simulink model "SYT_A23_mod"  (Simulink 5.1)
settings: Solver=ode5  SolverMode=SingleTasking  StartTime=0.0  StopTime=20.0  FixedStep=0.1  RelTol=1e-3
settings Model: LastModifiedBy=Sommer  BooleanDataType=on  ProdHWDeviceType=Microprocessor

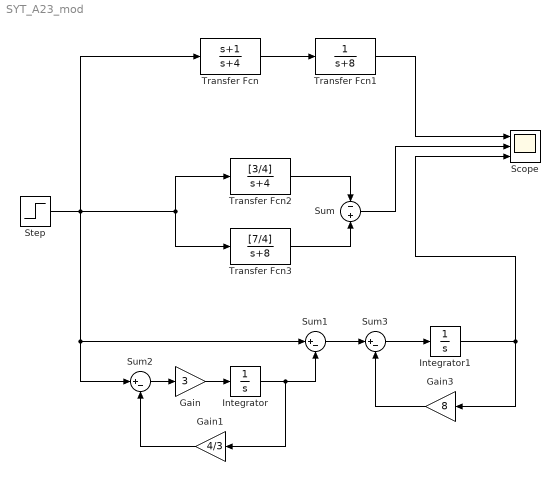
== system SYT_A23_mod ==
  Gain : Gain  Gain=3  SaturateOnIntegerOverflow=on
  Gain1 : Gain  Orientation=left  Gain=4/3  SaturateOnIntegerOverflow=on
  Gain3 : Gain  Orientation=left  Gain=8  SaturateOnIntegerOverflow=on
  Integrator : Integrator
  Integrator1 : Integrator
  Scope : Scope  NumInputPorts=3
      settings: YMin=-5~-5~-5  YMax=5~5~5
  Step : Step  SampleTime=0
  Sum : Sum  Inputs=-|+  SaturateOnIntegerOverflow=on  InputSameDT=on
  Sum1 : Sum  Inputs=|+-  SaturateOnIntegerOverflow=on  InputSameDT=on
  Sum2 : Sum  Inputs=|+-  SaturateOnIntegerOverflow=on  InputSameDT=on
  Sum3 : Sum  Inputs=|+-  SaturateOnIntegerOverflow=on  InputSameDT=on
  Transfer Fcn : TransferFcn  Numerator=[1 1]  Denominator=[1 4]
  Transfer Fcn1 : TransferFcn  Denominator=[1 8]
  Transfer Fcn2 : TransferFcn  Numerator=[3/4]  Denominator=[1 4]
  Transfer Fcn3 : TransferFcn  Numerator=[7/4]  Denominator=[1 8]
  wires:
  Transfer Fcn/1 -> Transfer Fcn1/1
  Step/1 -> Transfer Fcn/1, Transfer Fcn2/1, Transfer Fcn3/1, Sum2/1, Sum1/1
  Transfer Fcn1/1 -> Scope/1
  Transfer Fcn2/1 -> Sum/1
  Transfer Fcn3/1 -> Sum/2
  Sum/1 -> Scope/2
  Gain/1 -> Integrator/1
  Gain1/1 -> Sum2/2
  Sum2/1 -> Gain/1
  Integrator/1 -> Sum1/2, Gain1/1
  Sum3/1 -> Integrator1/1
  Gain3/1 -> Sum3/2
  Integrator1/1 -> Gain3/1, Scope/3
  Sum1/1 -> Sum3/1
